simulink model "sim1S"  (R2024a)
settings: Solver=VariableStepAuto  StartTime=0.0  StopTime=500  RelTol=1e-3
values from neighbouring files (symbols this model uses):
  den = cell2mat(den)    [sim1M.m]
  den_pp = cell2mat(den_pp)    [sim1M.m]
  den_proces = cell2mat(den_proces)    [sim1M.m]
  Kr = -0.33    [sim1M.m]    (also in sim2M.m = 1/(C*inv(B*Kn-A)*B))
  num = cell2mat(num)    [sim1M.m]
  num_pp = cell2mat(num_pp)    [sim1M.m]
  num_proces = cell2mat(num_proces)    [sim1M.m]
(part 1 of 3)
settings Model: Creator=grabo  LastModifiedBy=grabo
settings OptimizationCC: ReuseModelBlockBuffer=off
settings RTWCC: GPUComputeCapability=3.5

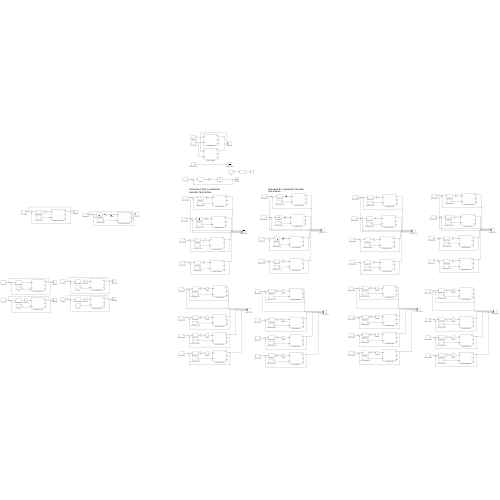
[thumbnail: Simulink's stored preview of the top-level diagram]
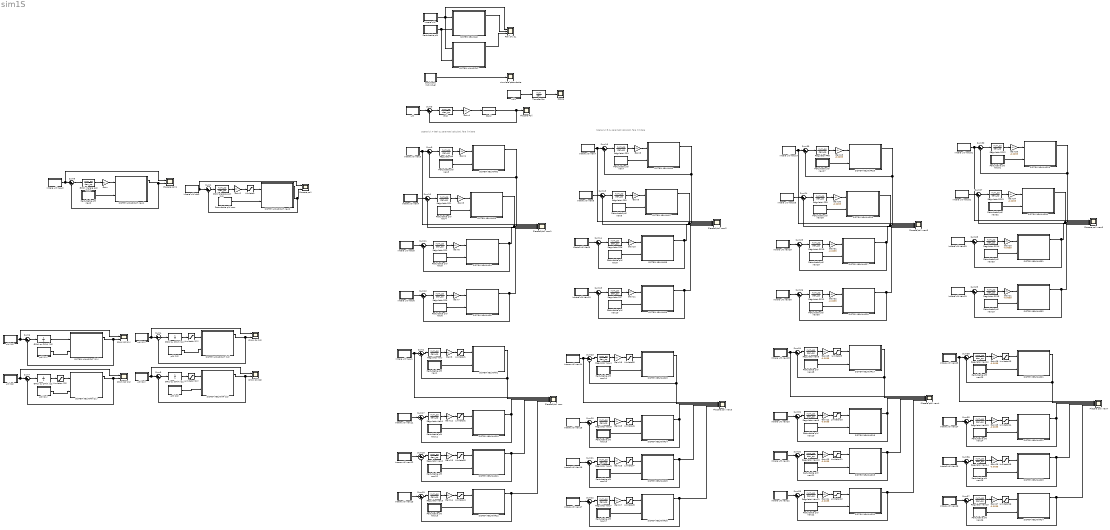
== system sim1S ==
  note: Scenariul A (G0) cu parametri calculati, fara limitare
  note: Scenariul B cu parametri calculati, fara limitare
  CMVK SL (11) : Scope  NumInputPorts=2
  CMVK SL (12) : Scope  NumInputPorts=2
  CMVK SN (21) : Scope  NumInputPorts=2
  CMVK SN (22) : Scope  NumInputPorts=2
  GR(s) cu CMVK (11) : TransferFcn  Numerator=1  Denominator=1
  GR(s) cu CMVK (12) : TransferFcn  Numerator=1  Denominator=1
  GR(s) cu CMVK (21) : TransferFcn  Numerator=1  Denominator=1
  GR(s) cu CMVK (22) : TransferFcn  Numerator=1  Denominator=1
  GR(s) plasare poli (12) : TransferFcn  Numerator=num_pp  Denominator=den_pp
  GR(s) plasare poli (12)1 : TransferFcn  Numerator=num_pp  Denominator=den_pp
  Gain{,1..18} (19 alike) : Gain  Gain=Kr
  Gain{19..34} (16 alike) : Gain  Gain=-0.0035
  Gp(s) : TransferFcn  Numerator=num_proces  Denominator=den_proces
  Gr(s) : TransferFcn  Numerator=num_pp  Denominator=den_pp
  Intrare u(t) : Subsystem  mask{With_u=1, Gref=80}
      mask prompts: With_u "With_u ="; Gref "Gref ="
  Intrare u(t) new : Subsystem  mask{With_u=1, Gref=80}
      mask prompts: With_u "With_u ="; Gref "Gref ="
  Intrare u(t) new1 : Subsystem  mask{With_u=1, Gref=80}
      mask prompts: With_u "With_u ="; Gref "Gref ="
  Intrare u(t) new10 : Subsystem  mask{With_u=1, Gref=80}
      mask prompts: With_u "With_u ="; Gref "Gref ="
  Intrare u(t) new11 : Subsystem  mask{With_u=1, Gref=80}
      mask prompts: With_u "With_u ="; Gref "Gref ="
  Intrare u(t) new12 : Subsystem  mask{With_u=1, Gref=80}
      mask prompts: With_u "With_u ="; Gref "Gref ="
  Intrare u(t) new13 : Subsystem  mask{With_u=1, Gref=80}
      mask prompts: With_u "With_u ="; Gref "Gref ="
  Intrare u(t) new14 : Subsystem  mask{With_u=1, Gref=80}
      mask prompts: With_u "With_u ="; Gref "Gref ="
  Intrare u(t) new15 : Subsystem  mask{With_u=1, Gref=80}
      mask prompts: With_u "With_u ="; Gref "Gref ="
  Intrare u(t) new16 : Subsystem  mask{With_u=1, Gref=80}
      mask prompts: With_u "With_u ="; Gref "Gref ="
  Intrare u(t) new17 : Subsystem  mask{With_u=1, Gref=80}
      mask prompts: With_u "With_u ="; Gref "Gref ="
  Intrare u(t) new18 : Subsystem  mask{With_u=1, Gref=80}
      mask prompts: With_u "With_u ="; Gref "Gref ="
  Intrare u(t) new19 : Subsystem  mask{With_u=1, Gref=80}
      mask prompts: With_u "With_u ="; Gref "Gref ="
  Intrare u(t) new2 : Subsystem  mask{With_u=1, Gref=80}
      mask prompts: With_u "With_u ="; Gref "Gref ="
  Intrare u(t) new20 : Subsystem  mask{With_u=1, Gref=80}
      mask prompts: With_u "With_u ="; Gref "Gref ="
  Intrare u(t) new21 : Subsystem  mask{With_u=1, Gref=80}
      mask prompts: With_u "With_u ="; Gref "Gref ="
  Intrare u(t) new22 : Subsystem  mask{With_u=1, Gref=80}
      mask prompts: With_u "With_u ="; Gref "Gref ="
  Intrare u(t) new23 : Subsystem  mask{With_u=1, Gref=80}
      mask prompts: With_u "With_u ="; Gref "Gref ="
  Intrare u(t) new24 : Subsystem  mask{With_u=1, Gref=80}
      mask prompts: With_u "With_u ="; Gref "Gref ="
  Intrare u(t) new25 : Subsystem  mask{With_u=1, Gref=80}
      mask prompts: With_u "With_u ="; Gref "Gref ="
  Intrare u(t) new26 : Subsystem  mask{With_u=1, Gref=80}
      mask prompts: With_u "With_u ="; Gref "Gref ="
  Intrare u(t) new27 : Subsystem  mask{With_u=1, Gref=80}
      mask prompts: With_u "With_u ="; Gref "Gref ="
  Intrare u(t) new28 : Subsystem  mask{With_u=1, Gref=80}
      mask prompts: With_u "With_u ="; Gref "Gref ="
  Intrare u(t) new29 : Subsystem  mask{With_u=1, Gref=80}
      mask prompts: With_u "With_u ="; Gref "Gref ="
  Intrare u(t) new3 : Subsystem  mask{With_u=1, Gref=80}
      mask prompts: With_u "With_u ="; Gref "Gref ="
  Intrare u(t) new30 : Subsystem  mask{With_u=1, Gref=80}
      mask prompts: With_u "With_u ="; Gref "Gref ="
  Intrare u(t) new31 : Subsystem  mask{With_u=1, Gref=80}
      mask prompts: With_u "With_u ="; Gref "Gref ="
  Intrare u(t) new32 : Subsystem  mask{With_u=1, Gref=80}
      mask prompts: With_u "With_u ="; Gref "Gref ="
  Intrare u(t) new33 : Subsystem  mask{With_u=1, Gref=80}
      mask prompts: With_u "With_u ="; Gref "Gref ="
  Intrare u(t) new4 : Subsystem  mask{With_u=1, Gref=80}
      mask prompts: With_u "With_u ="; Gref "Gref ="
  Intrare u(t) new5 : Subsystem  mask{With_u=1, Gref=80}
      mask prompts: With_u "With_u ="; Gref "Gref ="
  Intrare u(t) new6 : Subsystem  mask{With_u=1, Gref=80}
      mask prompts: With_u "With_u ="; Gref "Gref ="
  Intrare u(t) new7 : Subsystem  mask{With_u=1, Gref=80}
      mask prompts: With_u "With_u ="; Gref "Gref ="
  Intrare u(t) new8 : Subsystem  mask{With_u=1, Gref=80}
      mask prompts: With_u "With_u ="; Gref "Gref ="
  Intrare u(t) new9 : Subsystem  mask{With_u=1, Gref=80}
      mask prompts: With_u "With_u ="; Gref "Gref ="
  Limitator{,1..16} (17 alike) : Saturate  UpperLimit=500  LowerLimit=0
  Limitator (12) : Saturate  UpperLimit=500  LowerLimit=0
  Limitator (21) : Saturate  UpperLimit=500  LowerLimit=0
  Limitator (22) : Saturate  UpperLimit=500  LowerLimit=0
  Perturbatie p(t) : Subsystem  mask{Dg=100*10^3, Ag=0.8, tgM=40, With_p=1}
      mask prompts: Dg "Dg ="; Ag "Ag ="; tgM "tgM ="; With_p "With_p ="
  Perturbatie p(t) new : Subsystem  mask{Dg=100000, Ag=0.8, tgM=40, With_p=0}
      mask prompts: Dg "Dg ="; Ag "Ag ="; tgM "tgM ="; With_p "With_p ="
  Perturbatie p(t) new1 : Subsystem  mask{Dg=40*10^4, Ag=0.8, tgM=40, With_p=0}
      mask prompts: Dg "Dg ="; Ag "Ag ="; tgM "tgM ="; With_p "With_p ="
  Perturbatie p(t) new10 : Subsystem  mask{Dg=100*10^3, Ag=0.8, tgM=40, With_p=1}
      mask prompts: Dg "Dg ="; Ag "Ag ="; tgM "tgM ="; With_p "With_p ="
  Perturbatie p(t) new11 : Subsystem  mask{Dg=40*10^4, Ag=0.8, tgM=40, With_p=0}
      mask prompts: Dg "Dg ="; Ag "Ag ="; tgM "tgM ="; With_p "With_p ="
  Perturbatie p(t) new12 : Subsystem  mask{Dg=40*10^4, Ag=0.8, tgM=40, With_p=0}
      mask prompts: Dg "Dg ="; Ag "Ag ="; tgM "tgM ="; With_p "With_p ="
  Perturbatie p(t) new13 : Subsystem  mask{Dg=40*10^4, Ag=0.8, tgM=40, With_p=0}
      mask prompts: Dg "Dg ="; Ag "Ag ="; tgM "tgM ="; With_p "With_p ="
  Perturbatie p(t) new14 : Subsystem  mask{Dg=10*10^4, Ag=0.8, tgM=40, With_p=1}
      mask prompts: Dg "Dg ="; Ag "Ag ="; tgM "tgM ="; With_p "With_p ="
  Perturbatie p(t) new15 : Subsystem  mask{Dg=40*10^4, Ag=0.8, tgM=40, With_p=1}
      mask prompts: Dg "Dg ="; Ag "Ag ="; tgM "tgM ="; With_p "With_p ="
  Perturbatie p(t) new16 : Subsystem  mask{Dg=70*10^4, Ag=0.8, tgM=40, With_p=1}
      mask prompts: Dg "Dg ="; Ag "Ag ="; tgM "tgM ="; With_p "With_p ="
  Perturbatie p(t) new17 : Subsystem  mask{Dg=100*10^4, Ag=0.8, tgM=40, With_p=1}
      mask prompts: Dg "Dg ="; Ag "Ag ="; tgM "tgM ="; With_p "With_p ="
  Perturbatie p(t) new18 : Subsystem  mask{Dg=40*10^4, Ag=0.8, tgM=40, With_p=0}
      mask prompts: Dg "Dg ="; Ag "Ag ="; tgM "tgM ="; With_p "With_p ="
  Perturbatie p(t) new19 : Subsystem  mask{Dg=100*10^3, Ag=0.8, tgM=40, With_p=1}
      mask prompts: Dg "Dg ="; Ag "Ag ="; tgM "tgM ="; With_p "With_p ="
  Perturbatie p(t) new2 : Subsystem  mask{Dg=10*10^3, Ag=0.8, tgM=40, With_p=0}
      mask prompts: Dg "Dg ="; Ag "Ag ="; tgM "tgM ="; With_p "With_p ="
  Perturbatie p(t) new20 : Subsystem  mask{Dg=40*10^4, Ag=0.8, tgM=40, With_p=0}
      mask prompts: Dg "Dg ="; Ag "Ag ="; tgM "tgM ="; With_p "With_p ="
  Perturbatie p(t) new21 : Subsystem  mask{Dg=40*10^4, Ag=0.8, tgM=40, With_p=0}
      mask prompts: Dg "Dg ="; Ag "Ag ="; tgM "tgM ="; With_p "With_p ="
  Perturbatie p(t) new22 : Subsystem  mask{Dg=40*10^4, Ag=0.8, tgM=40, With_p=0}
      mask prompts: Dg "Dg ="; Ag "Ag ="; tgM "tgM ="; With_p "With_p ="
  Perturbatie p(t) new23 : Subsystem  mask{Dg=10*10^4, Ag=0.8, tgM=40, With_p=1}
      mask prompts: Dg "Dg ="; Ag "Ag ="; tgM "tgM ="; With_p "With_p ="
  Perturbatie p(t) new24 : Subsystem  mask{Dg=40*10^4, Ag=0.8, tgM=40, With_p=1}
      mask prompts: Dg "Dg ="; Ag "Ag ="; tgM "tgM ="; With_p "With_p ="
  Perturbatie p(t) new25 : Subsystem  mask{Dg=70*10^4, Ag=0.8, tgM=40, With_p=1}
      mask prompts: Dg "Dg ="; Ag "Ag ="; tgM "tgM ="; With_p "With_p ="
  Perturbatie p(t) new26 : Subsystem  mask{Dg=100*10^4, Ag=0.8, tgM=40, With_p=1}
      mask prompts: Dg "Dg ="; Ag "Ag ="; tgM "tgM ="; With_p "With_p ="
  Perturbatie p(t) new27 : Subsystem  mask{Dg=10*10^3, Ag=0.8, tgM=40, With_p=0}
      mask prompts: Dg "Dg ="; Ag "Ag ="; tgM "tgM ="; With_p "With_p ="
  Perturbatie p(t) new28 : Subsystem  mask{Dg=10*10^3, Ag=0.8, tgM=40, With_p=0}
      mask prompts: Dg "Dg ="; Ag "Ag ="; tgM "tgM ="; With_p "With_p ="
  Perturbatie p(t) new29 : Subsystem  mask{Dg=10*10^3, Ag=0.8, tgM=40, With_p=0}
      mask prompts: Dg "Dg ="; Ag "Ag ="; tgM "tgM ="; With_p "With_p ="
  Perturbatie p(t) new3 : Subsystem  mask{Dg=10*10^3, Ag=0.8, tgM=40, With_p=0}
      mask prompts: Dg "Dg ="; Ag "Ag ="; tgM "tgM ="; With_p "With_p ="
  Perturbatie p(t) new30 : Subsystem  mask{Dg=10*10^3, Ag=0.8, tgM=40, With_p=0}
      mask prompts: Dg "Dg ="; Ag "Ag ="; tgM "tgM ="; With_p "With_p ="
  Perturbatie p(t) new31 : Subsystem  mask{Dg=10*10^3, Ag=0.8, tgM=40, With_p=1}
      mask prompts: Dg "Dg ="; Ag "Ag ="; tgM "tgM ="; With_p "With_p ="
  Perturbatie p(t) new32 : Subsystem  mask{Dg=40*10^3, Ag=0.8, tgM=40, With_p=1}
      mask prompts: Dg "Dg ="; Ag "Ag ="; tgM "tgM ="; With_p "With_p ="
  Perturbatie p(t) new33 : Subsystem  mask{Dg=70*10^3, Ag=0.8, tgM=40, With_p=1}
      mask prompts: Dg "Dg ="; Ag "Ag ="; tgM "tgM ="; With_p "With_p ="
  Perturbatie p(t) new4 : Subsystem  mask{Dg=10*10^3, Ag=0.8, tgM=40, With_p=0}
      mask prompts: Dg "Dg ="; Ag "Ag ="; tgM "tgM ="; With_p "With_p ="
  Perturbatie p(t) new5 : Subsystem  mask{Dg=10*10^3, Ag=0.8, tgM=40, With_p=0}
      mask prompts: Dg "Dg ="; Ag "Ag ="; tgM "tgM ="; With_p "With_p ="
  Perturbatie p(t) new6 : Subsystem  mask{Dg=10*10^3, Ag=0.8, tgM=40, With_p=0}
      mask prompts: Dg "Dg ="; Ag "Ag ="; tgM "tgM ="; With_p "With_p ="
  Perturbatie p(t) new7 : Subsystem  mask{Dg=10*10^3, Ag=0.8, tgM=40, With_p=1}
      mask prompts: Dg "Dg ="; Ag "Ag ="; tgM "tgM ="; With_p "With_p ="
  Perturbatie p(t) new8 : Subsystem  mask{Dg=40*10^3, Ag=0.8, tgM=40, With_p=1}
      mask prompts: Dg "Dg ="; Ag "Ag ="; tgM "tgM ="; With_p "With_p ="
  Perturbatie p(t) new9 : Subsystem  mask{Dg=70*10^3, Ag=0.8, tgM=40, With_p=1}
      mask prompts: Dg "Dg ="; Ag "Ag ="; tgM "tgM ="; With_p "With_p ="
  Plasare Poli : Scope
  Plasare poli : Scope  NumInputPorts=2
  Plasare poli new{,1..7} (8 alike) : Scope  NumInputPorts=5
  Plasare poli1 : Scope  NumInputPorts=2
  "Ref, SN, SL" : Scope  NumInputPorts=3
  Regulator PP{,1..15} (16 alike) : TransferFcn  Numerator=num_pp  Denominator=den_pp
  Regulator new{,1..15} (16 alike) : TransferFcn  Numerator=num_pp  Denominator=den_pp
  SISTEM LINIARIZAT : Subsystem  mask{V=120, Ag=0.8, tgM=40, Xb=0.0054, Gb=80, p1=0.019, p2=0.021, p3=10.19*10^(-6), n=0.177, G0=300}
      mask prompts: V "V ="; Ag "Ag ="; tgM "tgM ="; Xb "Xb ="; Gb "Gb ="; p1 "p1 ="; p2 "p2 ="; p3 "p3 ="; n "n ="; G0 "G0 ="
  SISTEM LINIARIZAT (11) : Subsystem  mask{V=120, Ag=0.8, tgM=40, Xb=0.0054, Gb=80, p1=0.019, p2=0.021, p3=10.19*10^(-6), n=0.177, G0=150}
      mask prompts: V "V ="; Ag "Ag ="; tgM "tgM ="; Xb "Xb ="; Gb "Gb ="; p1 "p1 ="; p2 "p2 ="; p3 "p3 ="; n "n ="; G0 "G0 ="
  SISTEM LINIARIZAT (12) : Subsystem  mask{V=120, Ag=0.8, tgM=40, Xb=0.0054, Gb=80, p1=0.019, p2=0.021, p3=10.19*10^(-6), n=0.177, G0=150}
      mask prompts: V "V ="; Ag "Ag ="; tgM "tgM ="; Xb "Xb ="; Gb "Gb ="; p1 "p1 ="; p2 "p2 ="; p3 "p3 ="; n "n ="; G0 "G0 ="
  SISTEM LINIARIZAT new1 : Subsystem  mask{V=120, Ag=0.8, tgM=40, Xb=0.0054, Gb=80, p1=0.019, p2=0.021, p3=10.19*10^(-6), n=0.177, G0=150}
      mask prompts: V "V ="; Ag "Ag ="; tgM "tgM ="; Xb "Xb ="; Gb "Gb ="; p1 "p1 ="; p2 "p2 ="; p3 "p3 ="; n "n ="; G0 "G0 ="
  SISTEM LINIARIZAT new2 : Subsystem  mask{V=120, Ag=0.8, tgM=40, Xb=0.0054, Gb=80, p1=0.019, p2=0.021, p3=10.19*10^(-6), n=0.177, G0=350}
      mask prompts: V "V ="; Ag "Ag ="; tgM "tgM ="; Xb "Xb ="; Gb "Gb ="; p1 "p1 ="; p2 "p2 ="; p3 "p3 ="; n "n ="; G0 "G0 ="
  SISTEM NELINIAR : Subsystem  mask{V=120, Gb=80, p1=0.019, p2=0.021, p3=10.19*10^(-6), n=0.177, G0=300}
      mask prompts: V "V ="; Gb "Gb ="; p1 "p1 ="; p2 "p2 ="; p3 "p3 ="; n "n ="; G0 "G0 ="
  SISTEM NELINIAR (21) : Subsystem  mask{V=120, Gb=80, p1=0.019, p2=0.021, p3=10.19*10^(-6), n=0.177, G0=150}
      mask prompts: V "V ="; Gb "Gb ="; p1 "p1 ="; p2 "p2 ="; p3 "p3 ="; n "n ="; G0 "G0 ="
  SISTEM NELINIAR (22) : Subsystem  mask{V=120, Gb=80, p1=0.019, p2=0.021, p3=10.19*10^(-6), n=0.177, G0=150}
      mask prompts: V "V ="; Gb "Gb ="; p1 "p1 ="; p2 "p2 ="; p3 "p3 ="; n "n ="; G0 "G0 ="
  SISTEM NELINIAR1 : Subsystem  mask{V=120, Gb=80, p1=0.019, p2=0.021, p3=10.19*10^(-6), n=0.177, G0=150}
      mask prompts: V "V ="; Gb "Gb ="; p1 "p1 ="; p2 "p2 ="; p3 "p3 ="; n "n ="; G0 "G0 ="
  SISTEM NELINIAR10 : Subsystem  mask{V=120, Gb=80, p1=0.019, p2=0.021, p3=10.19*10^(-6), n=0.177, G0=200}
      mask prompts: V "V ="; Gb "Gb ="; p1 "p1 ="; p2 "p2 ="; p3 "p3 ="; n "n ="; G0 "G0 ="
  SISTEM NELINIAR11 : Subsystem  mask{V=120, Gb=80, p1=0.019, p2=0.021, p3=10.19*10^(-6), n=0.177, G0=250}
      mask prompts: V "V ="; Gb "Gb ="; p1 "p1 ="; p2 "p2 ="; p3 "p3 ="; n "n ="; G0 "G0 ="
  SISTEM NELINIAR12 : Subsystem  mask{V=120, Gb=80, p1=0.019, p2=0.021, p3=10.19*10^(-6), n=0.177, G0=300}
      mask prompts: V "V ="; Gb "Gb ="; p1 "p1 ="; p2 "p2 ="; p3 "p3 ="; n "n ="; G0 "G0 ="
  SISTEM NELINIAR13 : Subsystem  mask{V=120, Gb=80, p1=0.019, p2=0.021, p3=10.19*10^(-6), n=0.177, G0=150}
      mask prompts: V "V ="; Gb "Gb ="; p1 "p1 ="; p2 "p2 ="; p3 "p3 ="; n "n ="; G0 "G0 ="
  SISTEM NELINIAR14 : Subsystem  mask{V=120, Gb=80, p1=0.019, p2=0.021, p3=10.19*10^(-6), n=0.177, G0=150}
      mask prompts: V "V ="; Gb "Gb ="; p1 "p1 ="; p2 "p2 ="; p3 "p3 ="; n "n ="; G0 "G0 ="
  SISTEM NELINIAR15 : Subsystem  mask{V=120, Gb=80, p1=0.019, p2=0.021, p3=10.19*10^(-6), n=0.177, G0=150}
      mask prompts: V "V ="; Gb "Gb ="; p1 "p1 ="; p2 "p2 ="; p3 "p3 ="; n "n ="; G0 "G0 ="
  SISTEM NELINIAR16 : Subsystem  mask{V=120, Gb=80, p1=0.019, p2=0.021, p3=10.19*10^(-6), n=0.177, G0=150}
      mask prompts: V "V ="; Gb "Gb ="; p1 "p1 ="; p2 "p2 ="; p3 "p3 ="; n "n ="; G0 "G0 ="
  SISTEM NELINIAR17 : Subsystem  mask{V=120, Gb=80, p1=0.019, p2=0.021, p3=10.19*10^(-6), n=0.177, G0=150}
      mask prompts: V "V ="; Gb "Gb ="; p1 "p1 ="; p2 "p2 ="; p3 "p3 ="; n "n ="; G0 "G0 ="
  SISTEM NELINIAR18 : Subsystem  mask{V=120, Gb=80, p1=0.019, p2=0.021, p3=10.19*10^(-6), n=0.177, G0=200}
      mask prompts: V "V ="; Gb "Gb ="; p1 "p1 ="; p2 "p2 ="; p3 "p3 ="; n "n ="; G0 "G0 ="
  SISTEM NELINIAR19 : Subsystem  mask{V=120, Gb=80, p1=0.019, p2=0.021, p3=10.19*10^(-6), n=0.177, G0=250}
      mask prompts: V "V ="; Gb "Gb ="; p1 "p1 ="; p2 "p2 ="; p3 "p3 ="; n "n ="; G0 "G0 ="
  SISTEM NELINIAR2 : Subsystem  mask{V=120, Gb=80, p1=0.019, p2=0.021, p3=10.19*10^(-6), n=0.177, G0=150}
      mask prompts: V "V ="; Gb "Gb ="; p1 "p1 ="; p2 "p2 ="; p3 "p3 ="; n "n ="; G0 "G0 ="
  SISTEM NELINIAR20 : Subsystem  mask{V=120, Gb=80, p1=0.019, p2=0.021, p3=10.19*10^(-6), n=0.177, G0=300}
      mask prompts: V "V ="; Gb "Gb ="; p1 "p1 ="; p2 "p2 ="; p3 "p3 ="; n "n ="; G0 "G0 ="
  SISTEM NELINIAR21 : Subsystem  mask{V=120, Gb=80, p1=0.019, p2=0.021, p3=10.19*10^(-6), n=0.177, G0=150}
      mask prompts: V "V ="; Gb "Gb ="; p1 "p1 ="; p2 "p2 ="; p3 "p3 ="; n "n ="; G0 "G0 ="
  SISTEM NELINIAR22 : Subsystem  mask{V=120, Gb=80, p1=0.019, p2=0.021, p3=10.19*10^(-6), n=0.177, G0=150}
      mask prompts: V "V ="; Gb "Gb ="; p1 "p1 ="; p2 "p2 ="; p3 "p3 ="; n "n ="; G0 "G0 ="
  SISTEM NELINIAR23 : Subsystem  mask{V=120, Gb=80, p1=0.019, p2=0.021, p3=10.19*10^(-6), n=0.177, G0=150}
      mask prompts: V "V ="; Gb "Gb ="; p1 "p1 ="; p2 "p2 ="; p3 "p3 ="; n "n ="; G0 "G0 ="
  SISTEM NELINIAR24 : Subsystem  mask{V=120, Gb=80, p1=0.019, p2=0.021, p3=10.19*10^(-6), n=0.177, G0=150}
      mask prompts: V "V ="; Gb "Gb ="; p1 "p1 ="; p2 "p2 ="; p3 "p3 ="; n "n ="; G0 "G0 ="
  SISTEM NELINIAR25 : Subsystem  mask{V=120, Gb=80, p1=0.019, p2=0.021, p3=10.19*10^(-6), n=0.177, G0=150}
      mask prompts: V "V ="; Gb "Gb ="; p1 "p1 ="; p2 "p2 ="; p3 "p3 ="; n "n ="; G0 "G0 ="
  SISTEM NELINIAR26 : Subsystem  mask{V=120, Gb=80, p1=0.019, p2=0.021, p3=10.19*10^(-6), n=0.177, G0=200}
      mask prompts: V "V ="; Gb "Gb ="; p1 "p1 ="; p2 "p2 ="; p3 "p3 ="; n "n ="; G0 "G0 ="
  SISTEM NELINIAR27 : Subsystem  mask{V=120, Gb=80, p1=0.019, p2=0.021, p3=10.19*10^(-6), n=0.177, G0=250}
      mask prompts: V "V ="; Gb "Gb ="; p1 "p1 ="; p2 "p2 ="; p3 "p3 ="; n "n ="; G0 "G0 ="
  SISTEM NELINIAR28 : Subsystem  mask{V=120, Gb=80, p1=0.019, p2=0.021, p3=10.19*10^(-6), n=0.177, G0=300}
      mask prompts: V "V ="; Gb "Gb ="; p1 "p1 ="; p2 "p2 ="; p3 "p3 ="; n "n ="; G0 "G0 ="
  SISTEM NELINIAR29 : Subsystem  mask{V=120, Gb=80, p1=0.019, p2=0.021, p3=10.19*10^(-6), n=0.177, G0=150}
      mask prompts: V "V ="; Gb "Gb ="; p1 "p1 ="; p2 "p2 ="; p3 "p3 ="; n "n ="; G0 "G0 ="
  SISTEM NELINIAR3 : Subsystem  mask{V=120, Gb=80, p1=0.019, p2=0.021, p3=10.19*10^(-6), n=0.177, G0=200}
      mask prompts: V "V ="; Gb "Gb ="; p1 "p1 ="; p2 "p2 ="; p3 "p3 ="; n "n ="; G0 "G0 ="
  SISTEM NELINIAR30 : Subsystem  mask{V=120, Gb=80, p1=0.019, p2=0.021, p3=10.19*10^(-6), n=0.177, G0=200}
      mask prompts: V "V ="; Gb "Gb ="; p1 "p1 ="; p2 "p2 ="; p3 "p3 ="; n "n ="; G0 "G0 ="
  SISTEM NELINIAR31 : Subsystem  mask{V=120, Gb=80, p1=0.019, p2=0.021, p3=10.19*10^(-6), n=0.177, G0=250}
      mask prompts: V "V ="; Gb "Gb ="; p1 "p1 ="; p2 "p2 ="; p3 "p3 ="; n "n ="; G0 "G0 ="
  SISTEM NELINIAR32 : Subsystem  mask{V=120, Gb=80, p1=0.019, p2=0.021, p3=10.19*10^(-6), n=0.177, G0=300}
      mask prompts: V "V ="; Gb "Gb ="; p1 "p1 ="; p2 "p2 ="; p3 "p3 ="; n "n ="; G0 "G0 ="
  SISTEM NELINIAR4 : Subsystem  mask{V=120, Gb=80, p1=0.019, p2=0.021, p3=10.19*10^(-6), n=0.177, G0=250}
      mask prompts: V "V ="; Gb "Gb ="; p1 "p1 ="; p2 "p2 ="; p3 "p3 ="; n "n ="; G0 "G0 ="
  SISTEM NELINIAR5 : Subsystem  mask{V=120, Gb=80, p1=0.019, p2=0.021, p3=10.19*10^(-6), n=0.177, G0=300}
      mask prompts: V "V ="; Gb "Gb ="; p1 "p1 ="; p2 "p2 ="; p3 "p3 ="; n "n ="; G0 "G0 ="
  SISTEM NELINIAR6 : Subsystem  mask{V=120, Gb=80, p1=0.019, p2=0.021, p3=10.19*10^(-6), n=0.177, G0=150}
      mask prompts: V "V ="; Gb "Gb ="; p1 "p1 ="; p2 "p2 ="; p3 "p3 ="; n "n ="; G0 "G0 ="
  SISTEM NELINIAR7 : Subsystem  mask{V=120, Gb=80, p1=0.019, p2=0.021, p3=10.19*10^(-6), n=0.177, G0=200}
      mask prompts: V "V ="; Gb "Gb ="; p1 "p1 ="; p2 "p2 ="; p3 "p3 ="; n "n ="; G0 "G0 ="
  SISTEM NELINIAR8 : Subsystem  mask{V=120, Gb=80, p1=0.019, p2=0.021, p3=10.19*10^(-6), n=0.177, G0=250}
      mask prompts: V "V ="; Gb "Gb ="; p1 "p1 ="; p2 "p2 ="; p3 "p3 ="; n "n ="; G0 "G0 ="
  SISTEM NELINIAR9 : Subsystem  mask{V=120, Gb=80, p1=0.019, p2=0.021, p3=10.19*10^(-6), n=0.177, G0=300}
      mask prompts: V "V ="; Gb "Gb ="; p1 "p1 ="; p2 "p2 ="; p3 "p3 ="; n "n ="; G0 "G0 ="
  Scope : Scope
  Sum{1..39} (39 alike) : Sum  Inputs=|+-
  Transfer Fcn : TransferFcn  Numerator=num  Denominator=den
  p(t) (11) : Subsystem  mask{Dg=100000, Ag=0.8, tgM=40, With_p=0}
      mask prompts: Dg "Dg ="; Ag "Ag ="; tgM "tgM ="; With_p "With_p ="
  p(t) (12) : Subsystem  mask{Dg=100000, Ag=0.8, tgM=40, With_p=0}
      mask prompts: Dg "Dg ="; Ag "Ag ="; tgM "tgM ="; With_p "With_p ="
  p(t) (21) : Subsystem  mask{Dg=100000, Ag=0.8, tgM=40, With_p=0}
      mask prompts: Dg "Dg ="; Ag "Ag ="; tgM "tgM ="; With_p "With_p ="
  p(t) (22) : Subsystem  mask{Dg=100000, Ag=0.8, tgM=40, With_p=0}
      mask prompts: Dg "Dg ="; Ag "Ag ="; tgM "tgM ="; With_p "With_p ="
  pertubatie individual : Subsystem  mask{Dg=10*10^3, Ag=0.8, tgM=40}
      mask prompts: Dg "Dg ="; Ag "Ag ="; tgM "tgM ="
  simulare perturbatie : Scope
  u(t) : Subsystem  mask{With_u=1, Gref=80}
      mask prompts: With_u "With_u ="; Gref "Gref ="
  u(t) (11) : Subsystem  mask{With_u=1, Gref=80}
      mask prompts: With_u "With_u ="; Gref "Gref ="
  u(t) (12) : Subsystem  mask{With_u=1, Gref=80}
      mask prompts: With_u "With_u ="; Gref "Gref ="
  u(t) (21) : Subsystem  mask{With_u=1, Gref=80}
      mask prompts: With_u "With_u ="; Gref "Gref ="
  u(t) (22) : Subsystem  mask{With_u=1, Gref=80}
      mask prompts: With_u "With_u ="; Gref "Gref ="
  u(t)1 : Subsystem  mask{With_u=1, Gref=80}
      mask prompts: With_u "With_u ="; Gref "Gref ="
  wires:
  pertubatie individual/1(p(t)) -> simulare perturbatie/1
  Intrare u(t)/1(u(t)) -> SISTEM LINIARIZAT/1(u(t)), "Ref, SN, SL"/1, SISTEM NELINIAR/1(u(t))
  Perturbatie p(t)/1(p(t)) -> SISTEM LINIARIZAT/2(p(t)), SISTEM NELINIAR/2(p(t))
  Perturbatie p(t) new/1(p(t)) -> SISTEM LINIARIZAT new2/2(p(t))
  Intrare u(t) new/1(u(t)) -> Plasare poli/1, Sum1/1
  Sum1/1 -> GR(s) plasare poli (12)/1
  Sum2/1 -> Regulator new/1
  Perturbatie p(t) new1/1(p(t)) -> SISTEM NELINIAR1/2(p(t))
  Intrare u(t) new1/1(u(t)) -> Plasare poli new/1, Sum2/1
  SISTEM NELINIAR1/1(G(t)) -> Plasare poli new/2, Sum2/2
  Sum3/1 -> Gr(s)/1
  u(t)/1(u(t)) -> Sum3/1
  Gr(s)/1 -> Gain4/1
  Gp(s)/1 -> Sum3/2, Plasare Poli/1
  Regulator new/1 -> Gain3/1
  Limitator1/1 -> SISTEM NELINIAR1/1(u(t))
  GR(s) plasare poli (12)/1 -> Gain2/1
  Limitator/1 -> SISTEM LINIARIZAT new2/1(u(t))
  u(t) (22)/1(u(t)) -> CMVK SN (22)/1, Sum5/1
  p(t) (22)/1(p(t)) -> SISTEM NELINIAR (22)/2(p(t))
  Sum4/1 -> GR(s) cu CMVK (12)/1
  Sum5/1 -> GR(s) cu CMVK (22)/1
  SISTEM NELINIAR (22)/1(G(t)) -> Sum5/2, CMVK SN (22)/2
  u(t) (12)/1(u(t)) -> CMVK SL (12)/1, Sum4/1
  SISTEM LINIARIZAT (12)/1(G(t)) -> Sum4/2, CMVK SL (12)/2
  p(t) (12)/1(p(t)) -> SISTEM LINIARIZAT (12)/2(p(t))
  GR(s) cu CMVK (12)/1 -> Limitator (12)/1
  Limitator (12)/1 -> SISTEM LINIARIZAT (12)/1(u(t))
  GR(s) cu CMVK (22)/1 -> Limitator (22)/1
  Limitator (22)/1 -> SISTEM NELINIAR (22)/1(u(t))
  GR(s) cu CMVK (11)/1 -> SISTEM LINIARIZAT (11)/1(u(t))
  Sum6/1 -> GR(s) cu CMVK (11)/1
  SISTEM LINIARIZAT (11)/1(G(t)) -> Sum6/2, CMVK SL (11)/2
  u(t) (11)/1(u(t)) -> CMVK SL (11)/1, Sum6/1
  p(t) (11)/1(p(t)) -> SISTEM LINIARIZAT (11)/2(p(t))
  Limitator (21)/1 -> SISTEM NELINIAR (21)/1(u(t))
  GR(s) cu CMVK (21)/1 -> Limitator (21)/1
  u(t) (21)/1(u(t)) -> CMVK SN (21)/1, Sum7/1
  Sum7/1 -> GR(s) cu CMVK (21)/1
  p(t) (21)/1(p(t)) -> SISTEM NELINIAR (21)/2(p(t))
  SISTEM NELINIAR (21)/1(G(t)) -> Sum7/2, CMVK SN (21)/2
  GR(s) plasare poli (12)1/1 -> Gain/1
  Intrare u(t) new2/1(u(t)) -> Plasare poli1/1, Sum8/1
  Sum8/1 -> GR(s) plasare poli (12)1/1
  SISTEM LINIARIZAT new1/1(G(t)) -> Sum8/2, Plasare poli1/2
  Perturbatie p(t) new2/1(p(t)) -> SISTEM LINIARIZAT new1/2(p(t))
  Regulator PP/1 -> Gain1/1
  Perturbatie p(t) new3/1(p(t)) -> SISTEM NELINIAR2/2(p(t))
  Intrare u(t) new3/1(u(t)) -> Plasare poli new1/1, Sum9/1
  Sum9/1 -> Regulator PP/1
  SISTEM NELINIAR2/1(G(t)) -> Sum9/2, Plasare poli new1/2
  Gain/1 -> SISTEM LINIARIZAT new1/1(u(t))
  Gain1/1 -> SISTEM NELINIAR2/1(u(t))
  Gain2/1 -> Limitator/1
  Gain3/1 -> Limitator1/1
  SISTEM LINIARIZAT new2/1(G(t)) -> Sum1/2, Plasare poli/2
  Gain4/1 -> Gp(s)/1
  SISTEM NELINIAR/1(G(t)) -> "Ref, SN, SL"/2
  SISTEM LINIARIZAT/1(G(t)) -> "Ref, SN, SL"/3
  Perturbatie p(t) new4/1(p(t)) -> SISTEM NELINIAR3/2(p(t))
  Gain5/1 -> SISTEM NELINIAR3/1(u(t))
  SISTEM NELINIAR3/1(G(t)) -> Sum10/2, Plasare poli new1/3
  Intrare u(t) new4/1(u(t)) -> Sum10/1
  Regulator PP1/1 -> Gain5/1
  Sum10/1 -> Regulator PP1/1
  Perturbatie p(t) new5/1(p(t)) -> SISTEM NELINIAR4/2(p(t))
  Gain6/1 -> SISTEM NELINIAR4/1(u(t))
  SISTEM NELINIAR4/1(G(t)) -> Plasare poli new1/4, Sum11/2
  Intrare u(t) new5/1(u(t)) -> Sum11/1
  Regulator PP2/1 -> Gain6/1
  Sum11/1 -> Regulator PP2/1
  Perturbatie p(t) new6/1(p(t)) -> SISTEM NELINIAR5/2(p(t))
  Gain7/1 -> SISTEM NELINIAR5/1(u(t))
  SISTEM NELINIAR5/1(G(t)) -> Plasare poli new1/5, Sum12/2
  Intrare u(t) new6/1(u(t)) -> Sum12/1
  Regulator PP3/1 -> Gain7/1
  Sum12/1 -> Regulator PP3/1
  Sum14/1 -> Regulator PP6/1
  Regulator PP6/1 -> Gain10/1
  SISTEM NELINIAR8/1(G(t)) -> Plasare poli new2/4, Sum14/2
  Intrare u(t) new8/1(u(t)) -> Sum13/1
  Sum13/1 -> Regulator PP5/1
  Regulator PP5/1 -> Gain9/1
  Gain9/1 -> SISTEM NELINIAR7/1(u(t))
  Perturbatie p(t) new8/1(p(t)) -> SISTEM NELINIAR7/2(p(t))
  Gain10/1 -> SISTEM NELINIAR8/1(u(t))
  Regulator PP7/1 -> Gain11/1
  Sum15/1 -> Regulator PP7/1
  Intrare u(t) new9/1(u(t)) -> Sum14/1
  Intrare u(t) new10/1(u(t)) -> Sum15/1
  Perturbatie p(t) new9/1(p(t)) -> SISTEM NELINIAR8/2(p(t))
  SISTEM NELINIAR9/1(G(t)) -> Plasare poli new2/5, Sum15/2
  Gain11/1 -> SISTEM NELINIAR9/1(u(t))
  Perturbatie p(t) new7/1(p(t)) -> SISTEM NELINIAR6/2(p(t))
  Gain8/1 -> SISTEM NELINIAR6/1(u(t))
  SISTEM NELINIAR6/1(G(t)) -> Sum16/2, Plasare poli new2/2
  Intrare u(t) new7/1(u(t)) -> Plasare poli new2/1, Sum16/1
  SISTEM NELINIAR7/1(G(t)) -> Sum13/2, Plasare poli new2/3
  Regulator PP4/1 -> Gain8/1
  Perturbatie p(t) new10/1(p(t)) -> SISTEM NELINIAR9/2(p(t))
  Sum16/1 -> Regulator PP4/1
  SISTEM NELINIAR10/1(G(t)) -> Sum17/2, Plasare poli new/3
  Regulator new1/1 -> Gain12/1
  Sum17/1 -> Regulator new1/1
  Limitator2/1 -> SISTEM NELINIAR10/1(u(t))
  Gain12/1 -> Limitator2/1
  Intrare u(t) new11/1(u(t)) -> Sum17/1
  Perturbatie p(t) new11/1(p(t)) -> SISTEM NELINIAR10/2(p(t))
  Perturbatie p(t) new12/1(p(t)) -> SISTEM NELINIAR11/2(p(t))
  Gain13/1 -> Limitator3/1
  Regulator new2/1 -> Gain13/1
  Limitator3/1 -> SISTEM NELINIAR11/1(u(t))
  Sum18/1 -> Regulator new2/1
  Intrare u(t) new12/1(u(t)) -> Sum18/1
  SISTEM NELINIAR11/1(G(t)) -> Plasare poli new/4, Sum18/2
  Perturbatie p(t) new13/1(p(t)) -> SISTEM NELINIAR12/2(p(t))
  Gain14/1 -> Limitator4/1
  Regulator new3/1 -> Gain14/1
  Limitator4/1 -> SISTEM NELINIAR12/1(u(t))
  Sum19/1 -> Regulator new3/1
  Intrare u(t) new13/1(u(t)) -> Sum19/1
  SISTEM NELINIAR12/1(G(t)) -> Plasare poli new/5, Sum19/2
  Sum22/1 -> Regulator new7/1
  Intrare u(t) new17/1(u(t)) -> Sum22/1
  Regulator new7/1 -> Gain17/1
  Gain17/1 -> Limitator8/1
  Intrare u(t) new15/1(u(t)) -> Sum20/1
  Sum20/1 -> Regulator new5/1
  Gain15/1 -> Limitator6/1
  Regulator new5/1 -> Gain15/1
  Limitator6/1 -> SISTEM NELINIAR14/1(u(t))
  SISTEM NELINIAR14/1(G(t)) -> Sum20/2, Plasare poli new3/3
  Gain16/1 -> Limitator7/1
  Intrare u(t) new16/1(u(t)) -> Sum21/1
  SISTEM NELINIAR15/1(G(t)) -> Plasare poli new3/4, Sum21/2
  Sum21/1 -> Regulator new6/1
  Limitator7/1 -> SISTEM NELINIAR15/1(u(t))
  Regulator new6/1 -> Gain16/1
  Perturbatie p(t) new17/1(p(t)) -> SISTEM NELINIAR16/2(p(t))
  SISTEM NELINIAR16/1(G(t)) -> Plasare poli new3/5, Sum22/2
  Perturbatie p(t) new15/1(p(t)) -> SISTEM NELINIAR14/2(p(t))
  SISTEM NELINIAR13/1(G(t)) -> Plasare poli new3/2, Sum23/2
  Regulator new4/1 -> Gain18/1
  Sum23/1 -> Regulator new4/1
  Limitator5/1 -> SISTEM NELINIAR13/1(u(t))
  Limitator8/1 -> SISTEM NELINIAR16/1(u(t))
  Perturbatie p(t) new16/1(p(t)) -> SISTEM NELINIAR15/2(p(t))
  Gain18/1 -> Limitator5/1
  Intrare u(t) new14/1(u(t)) -> Plasare poli new3/1, Sum23/1
  Perturbatie p(t) new14/1(p(t)) -> SISTEM NELINIAR13/2(p(t))
  Sum33/1 -> Regulator new11/1
  Intrare u(t) new22/1(u(t)) -> Sum33/1
  Perturbatie p(t) new22/1(p(t)) -> SISTEM NELINIAR20/2(p(t))
  Perturbatie p(t) new20/1(p(t)) -> SISTEM NELINIAR18/2(p(t))
  Intrare u(t) new20/1(u(t)) -> Sum31/1
  Sum31/1 -> Regulator new9/1
  Regulator new9/1 -> Gain22/1
  Limitator10/1 -> SISTEM NELINIAR18/1(u(t))
  SISTEM NELINIAR18/1(G(t)) -> Sum31/2, Plasare poli new4/3
  Regulator new12/1 -> Gain28/1
  SISTEM NELINIAR21/1(G(t)) -> Plasare poli new7/2, Sum38/2
  Sum38/1 -> Regulator new12/1
  Limitator13/1 -> SISTEM NELINIAR21/1(u(t))
  Perturbatie p(t) new25/1(p(t)) -> SISTEM NELINIAR23/2(p(t))
  Limitator16/1 -> SISTEM NELINIAR24/1(u(t))
  Gain28/1 -> Limitator13/1
  Gain24/1 -> Limitator12/1
  SISTEM NELINIAR24/1(G(t)) -> Plasare poli new7/5, Sum37/2
  Perturbatie p(t) new26/1(p(t)) -> SISTEM NELINIAR24/2(p(t))
  Perturbatie p(t) new24/1(p(t)) -> SISTEM NELINIAR22/2(p(t))
  Sum36/1 -> Regulator new14/1
  Gain26/1 -> Limitator15/1
  SISTEM NELINIAR23/1(G(t)) -> Plasare poli new7/4, Sum36/2
  Intrare u(t) new25/1(u(t)) -> Sum36/1
  Limitator14/1 -> SISTEM NELINIAR22/1(u(t))
  SISTEM NELINIAR22/1(G(t)) -> Sum35/2, Plasare poli new7/3
  Regulator new13/1 -> Gain25/1
  Gain27/1 -> Limitator16/1
  Sum37/1 -> Regulator new15/1
  Intrare u(t) new24/1(u(t)) -> Sum35/1
  Gain22/1 -> Limitator10/1
  Regulator new15/1 -> Gain27/1
  Intrare u(t) new23/1(u(t)) -> Plasare poli new7/1, Sum38/1
  Perturbatie p(t) new23/1(p(t)) -> SISTEM NELINIAR21/2(p(t))
  Perturbatie p(t) new21/1(p(t)) -> SISTEM NELINIAR19/2(p(t))
  Intrare u(t) new21/1(u(t)) -> Sum32/1
  SISTEM NELINIAR19/1(G(t)) -> Plasare poli new4/4, Sum32/2
  Limitator11/1 -> SISTEM NELINIAR19/1(u(t))
  Perturbatie p(t) new19/1(p(t)) -> SISTEM NELINIAR32/2(p(t))
  Sum30/1 -> Regulator PP12/1
  Regulator PP12/1 -> Gain33/1
  Intrare u(t) new31/1(u(t)) -> Plasare poli new6/1, Sum30/1
  SISTEM NELINIAR30/1(G(t)) -> Sum27/2, Plasare poli new6/3
  Gain21/1 -> SISTEM NELINIAR32/1(u(t))
  SISTEM NELINIAR32/1(G(t)) -> Plasare poli new6/5, Sum29/2
  Gain33/1 -> SISTEM NELINIAR29/1(u(t))
  SISTEM NELINIAR29/1(G(t)) -> Sum30/2, Plasare poli new6/2
  Intrare u(t) new26/1(u(t)) -> Sum37/1
  Perturbatie p(t) new33/1(p(t)) -> SISTEM NELINIAR31/2(p(t))
  Regulator PP15/1 -> Gain21/1
  Perturbatie p(t) new32/1(p(t)) -> SISTEM NELINIAR30/2(p(t))
  Sum29/1 -> Regulator PP15/1
  Intrare u(t) new32/1(u(t)) -> Sum27/1
  Regulator new10/1 -> Gain23/1
  Regulator PP13/1 -> Gain34/1
  Sum27/1 -> Regulator PP13/1
  Regulator new11/1 -> Gain24/1
  SISTEM NELINIAR31/1(G(t)) -> Plasare poli new6/4, Sum28/2
  Regulator PP14/1 -> Gain20/1
  Intrare u(t) new19/1(u(t)) -> Sum29/1
  Sum25/1 -> Regulator PP10/1
  Regulator PP10/1 -> Gain31/1
  Intrare u(t) new28/1(u(t)) -> Sum24/1
  Sum24/1 -> Regulator PP9/1
  Regulator new14/1 -> Gain26/1
  Gain34/1 -> SISTEM NELINIAR30/1(u(t))
  Gain23/1 -> Limitator11/1
  Gain20/1 -> SISTEM NELINIAR31/1(u(t))
  Regulator PP9/1 -> Gain30/1
  Gain30/1 -> SISTEM NELINIAR26/1(u(t))
  Limitator15/1 -> SISTEM NELINIAR23/1(u(t))
  Perturbatie p(t) new28/1(p(t)) -> SISTEM NELINIAR26/2(p(t))
  Intrare u(t) new33/1(u(t)) -> Sum28/1
  SISTEM NELINIAR20/1(G(t)) -> Plasare poli new4/5, Sum33/2
  Gain31/1 -> SISTEM NELINIAR27/1(u(t))
  Regulator PP11/1 -> Gain32/1
  Sum26/1 -> Regulator PP11/1
  Intrare u(t) new29/1(u(t)) -> Sum25/1
  Intrare u(t) new30/1(u(t)) -> Sum26/1
  Perturbatie p(t) new29/1(p(t)) -> SISTEM NELINIAR27/2(p(t))
  SISTEM NELINIAR28/1(G(t)) -> Plasare poli new5/5, Sum26/2
  Perturbatie p(t) new27/1(p(t)) -> SISTEM NELINIAR25/2(p(t))
  SISTEM NELINIAR17/1(G(t)) -> Plasare poli new4/2, Sum34/2
  Perturbatie p(t) new31/1(p(t)) -> SISTEM NELINIAR29/2(p(t))
  Gain32/1 -> SISTEM NELINIAR28/1(u(t))
  Gain25/1 -> Limitator14/1
  Gain29/1 -> Limitator9/1
  SISTEM NELINIAR25/1(G(t)) -> Sum39/2, Plasare poli new5/2
  Gain19/1 -> SISTEM NELINIAR25/1(u(t))
  Intrare u(t) new27/1(u(t)) -> Plasare poli new5/1, Sum39/1
  SISTEM NELINIAR26/1(G(t)) -> Sum24/2, Plasare poli new5/3
  Regulator PP8/1 -> Gain19/1
  Sum32/1 -> Regulator new10/1
  Perturbatie p(t) new30/1(p(t)) -> SISTEM NELINIAR28/2(p(t))
  Sum39/1 -> Regulator PP8/1
  Regulator new8/1 -> Gain29/1
  Sum34/1 -> Regulator new8/1
  Limitator9/1 -> SISTEM NELINIAR17/1(u(t))
  Sum28/1 -> Regulator PP14/1
  Limitator12/1 -> SISTEM NELINIAR20/1(u(t))
  Sum35/1 -> Regulator new13/1
  Intrare u(t) new18/1(u(t)) -> Plasare poli new4/1, Sum34/1
  SISTEM NELINIAR27/1(G(t)) -> Plasare poli new5/4, Sum25/2
  Perturbatie p(t) new18/1(p(t)) -> SISTEM NELINIAR17/2(p(t))
  Transfer Fcn/1 -> Scope/1
  u(t)1/1(u(t)) -> Transfer Fcn/1

== system sim1S/Intrare u(t) ==
  Gain : Gain  Gain=With_u
  Step : Step  Time=0  After=Gref  SampleTime=0
  u(t) : Outport
  wires:
  Step/1 -> Gain/1
  Gain/1 -> u(t)/1

== system sim1S/Intrare u(t) new ==
  Gain : Gain  Gain=With_u
  Step : Step  Time=0  After=Gref  SampleTime=0
  u(t) : Outport
  wires:
  Step/1 -> Gain/1
  Gain/1 -> u(t)/1

== system sim1S/Intrare u(t) new1 ==
  Gain : Gain  Gain=With_u
  Step : Step  Time=0  After=Gref  SampleTime=0
  u(t) : Outport
  wires:
  Step/1 -> Gain/1
  Gain/1 -> u(t)/1

== system sim1S/Intrare u(t) new10 ==
  Gain : Gain  Gain=With_u
  Step : Step  Time=0  After=Gref  SampleTime=0
  u(t) : Outport
  wires:
  Step/1 -> Gain/1
  Gain/1 -> u(t)/1

== system sim1S/Intrare u(t) new11 ==
  Gain : Gain  Gain=With_u
  Step : Step  Time=0  After=Gref  SampleTime=0
  u(t) : Outport
  wires:
  Step/1 -> Gain/1
  Gain/1 -> u(t)/1

== system sim1S/Intrare u(t) new12 ==
  Gain : Gain  Gain=With_u
  Step : Step  Time=0  After=Gref  SampleTime=0
  u(t) : Outport
  wires:
  Step/1 -> Gain/1
  Gain/1 -> u(t)/1

== system sim1S/Intrare u(t) new13 ==
  Gain : Gain  Gain=With_u
  Step : Step  Time=0  After=Gref  SampleTime=0
  u(t) : Outport
  wires:
  Step/1 -> Gain/1
  Gain/1 -> u(t)/1

== system sim1S/Intrare u(t) new14 ==
  Gain : Gain  Gain=With_u
  Step : Step  Time=0  After=Gref  SampleTime=0
  u(t) : Outport
  wires:
  Step/1 -> Gain/1
  Gain/1 -> u(t)/1

== system sim1S/Intrare u(t) new15 ==
  Gain : Gain  Gain=With_u
  Step : Step  Time=0  After=Gref  SampleTime=0
  u(t) : Outport
  wires:
  Step/1 -> Gain/1
  Gain/1 -> u(t)/1

== system sim1S/Intrare u(t) new16 ==
  Gain : Gain  Gain=With_u
  Step : Step  Time=0  After=Gref  SampleTime=0
  u(t) : Outport
  wires:
  Step/1 -> Gain/1
  Gain/1 -> u(t)/1

== system sim1S/Intrare u(t) new17 ==
  Gain : Gain  Gain=With_u
  Step : Step  Time=0  After=Gref  SampleTime=0
  u(t) : Outport
  wires:
  Step/1 -> Gain/1
  Gain/1 -> u(t)/1

== system sim1S/Intrare u(t) new18 ==
  Gain : Gain  Gain=With_u
  Step : Step  Time=0  After=Gref  SampleTime=0
  u(t) : Outport
  wires:
  Step/1 -> Gain/1
  Gain/1 -> u(t)/1

== system sim1S/Intrare u(t) new19 ==
  Gain : Gain  Gain=With_u
  Step : Step  Time=0  After=Gref  SampleTime=0
  u(t) : Outport
  wires:
  Step/1 -> Gain/1
  Gain/1 -> u(t)/1

== system sim1S/Intrare u(t) new2 ==
  Gain : Gain  Gain=With_u
  Step : Step  Time=0  After=Gref  SampleTime=0
  u(t) : Outport
  wires:
  Step/1 -> Gain/1
  Gain/1 -> u(t)/1

== system sim1S/Intrare u(t) new20 ==
  Gain : Gain  Gain=With_u
  Step : Step  Time=0  After=Gref  SampleTime=0
  u(t) : Outport
  wires:
  Step/1 -> Gain/1
  Gain/1 -> u(t)/1

== system sim1S/Intrare u(t) new21 ==
  Gain : Gain  Gain=With_u
  Step : Step  Time=0  After=Gref  SampleTime=0
  u(t) : Outport
  wires:
  Step/1 -> Gain/1
  Gain/1 -> u(t)/1

== system sim1S/Intrare u(t) new22 ==
  Gain : Gain  Gain=With_u
  Step : Step  Time=0  After=Gref  SampleTime=0
  u(t) : Outport
  wires:
  Step/1 -> Gain/1
  Gain/1 -> u(t)/1

== system sim1S/Intrare u(t) new23 ==
  Gain : Gain  Gain=With_u
  Step : Step  Time=0  After=Gref  SampleTime=0
  u(t) : Outport
  wires:
  Step/1 -> Gain/1
  Gain/1 -> u(t)/1

== system sim1S/Intrare u(t) new24 ==
  Gain : Gain  Gain=With_u
  Step : Step  Time=0  After=Gref  SampleTime=0
  u(t) : Outport
  wires:
  Step/1 -> Gain/1
  Gain/1 -> u(t)/1

== system sim1S/Intrare u(t) new25 ==
  Gain : Gain  Gain=With_u
  Step : Step  Time=0  After=Gref  SampleTime=0
  u(t) : Outport
  wires:
  Step/1 -> Gain/1
  Gain/1 -> u(t)/1

== system sim1S/Intrare u(t) new26 ==
  Gain : Gain  Gain=With_u
  Step : Step  Time=0  After=Gref  SampleTime=0
  u(t) : Outport
  wires:
  Step/1 -> Gain/1
  Gain/1 -> u(t)/1

== system sim1S/Intrare u(t) new27 ==
  Gain : Gain  Gain=With_u
  Step : Step  Time=0  After=Gref  SampleTime=0
  u(t) : Outport
  wires:
  Step/1 -> Gain/1
  Gain/1 -> u(t)/1

== system sim1S/Intrare u(t) new28 ==
  Gain : Gain  Gain=With_u
  Step : Step  Time=0  After=Gref  SampleTime=0
  u(t) : Outport
  wires:
  Step/1 -> Gain/1
  Gain/1 -> u(t)/1

== system sim1S/Intrare u(t) new29 ==
  Gain : Gain  Gain=With_u
  Step : Step  Time=0  After=Gref  SampleTime=0
  u(t) : Outport
  wires:
  Step/1 -> Gain/1
  Gain/1 -> u(t)/1

== system sim1S/Intrare u(t) new3 ==
  Gain : Gain  Gain=With_u
  Step : Step  Time=0  After=Gref  SampleTime=0
  u(t) : Outport
  wires:
  Step/1 -> Gain/1
  Gain/1 -> u(t)/1

== system sim1S/Intrare u(t) new30 ==
  Gain : Gain  Gain=With_u
  Step : Step  Time=0  After=Gref  SampleTime=0
  u(t) : Outport
  wires:
  Step/1 -> Gain/1
  Gain/1 -> u(t)/1

== system sim1S/Intrare u(t) new31 ==
  Gain : Gain  Gain=With_u
  Step : Step  Time=0  After=Gref  SampleTime=0
  u(t) : Outport
  wires:
  Step/1 -> Gain/1
  Gain/1 -> u(t)/1

== system sim1S/Intrare u(t) new32 ==
  Gain : Gain  Gain=With_u
  Step : Step  Time=0  After=Gref  SampleTime=0
  u(t) : Outport
  wires:
  Step/1 -> Gain/1
  Gain/1 -> u(t)/1

== system sim1S/Intrare u(t) new33 ==
  Gain : Gain  Gain=With_u
  Step : Step  Time=0  After=Gref  SampleTime=0
  u(t) : Outport
  wires:
  Step/1 -> Gain/1
  Gain/1 -> u(t)/1

== system sim1S/Intrare u(t) new4 ==
  Gain : Gain  Gain=With_u
  Step : Step  Time=0  After=Gref  SampleTime=0
  u(t) : Outport
  wires:
  Step/1 -> Gain/1
  Gain/1 -> u(t)/1

== system sim1S/Intrare u(t) new5 ==
  Gain : Gain  Gain=With_u
  Step : Step  Time=0  After=Gref  SampleTime=0
  u(t) : Outport
  wires:
  Step/1 -> Gain/1
  Gain/1 -> u(t)/1

== system sim1S/Intrare u(t) new6 ==
  Gain : Gain  Gain=With_u
  Step : Step  Time=0  After=Gref  SampleTime=0
  u(t) : Outport
  wires:
  Step/1 -> Gain/1
  Gain/1 -> u(t)/1

== system sim1S/Intrare u(t) new7 ==
  Gain : Gain  Gain=With_u
  Step : Step  Time=0  After=Gref  SampleTime=0
  u(t) : Outport
  wires:
  Step/1 -> Gain/1
  Gain/1 -> u(t)/1

== system sim1S/Intrare u(t) new8 ==
  Gain : Gain  Gain=With_u
  Step : Step  Time=0  After=Gref  SampleTime=0
  u(t) : Outport
  wires:
  Step/1 -> Gain/1
  Gain/1 -> u(t)/1

== system sim1S/Intrare u(t) new9 ==
  Gain : Gain  Gain=With_u
  Step : Step  Time=0  After=Gref  SampleTime=0
  u(t) : Outport
  wires:
  Step/1 -> Gain/1
  Gain/1 -> u(t)/1

== system sim1S/Perturbatie p(t) ==
  Clock1 : Clock
  Constant1 : Constant  Value=Dg
  Constant2 : Constant  Value=Ag
  Constant3 : Constant  Value=-1/tgM
  Constant4 : Constant  Value=1/(tgM^2)
  Gain : Gain  Gain=With_p
  Math Function : Math  SignedPower=on
  Product1 : Product
  Product3 : Product  Inputs=5
  p(t) : Outport
  wires:
  Clock1/1 -> Product3/5, Product1/1
  Constant3/1 -> Product1/2
  Product1/1 -> Math Function/1
  Constant4/1 -> Product3/4
  Constant1/1 -> Product3/1
  Constant2/1 -> Product3/2
  Math Function/1 -> Product3/3
  Product3/1 -> Gain/1
  Gain/1 -> p(t)/1

== system sim1S/Perturbatie p(t) new ==
  Clock1 : Clock
  Constant1 : Constant  Value=Dg
  Constant2 : Constant  Value=Ag
  Constant3 : Constant  Value=-1/tgM
  Constant4 : Constant  Value=1/(tgM^2)
  Gain : Gain  Gain=With_p
  Math Function : Math  SignedPower=on
  Product1 : Product
  Product3 : Product  Inputs=5
  p(t) : Outport
  wires:
  Clock1/1 -> Product3/5, Product1/1
  Constant3/1 -> Product1/2
  Product1/1 -> Math Function/1
  Constant4/1 -> Product3/4
  Constant1/1 -> Product3/1
  Constant2/1 -> Product3/2
  Math Function/1 -> Product3/3
  Product3/1 -> Gain/1
  Gain/1 -> p(t)/1

== system sim1S/Perturbatie p(t) new1 ==
  Clock1 : Clock
  Constant1 : Constant  Value=Dg
  Constant2 : Constant  Value=Ag
  Constant3 : Constant  Value=-1/tgM
  Constant4 : Constant  Value=1/(tgM^2)
  Gain : Gain  Gain=With_p
  Math Function : Math  SignedPower=on
  Product1 : Product
  Product3 : Product  Inputs=5
  p(t) : Outport
  wires:
  Clock1/1 -> Product3/5, Product1/1
  Constant3/1 -> Product1/2
  Product1/1 -> Math Function/1
  Constant4/1 -> Product3/4
  Constant1/1 -> Product3/1
  Constant2/1 -> Product3/2
  Math Function/1 -> Product3/3
  Product3/1 -> Gain/1
  Gain/1 -> p(t)/1

== system sim1S/Perturbatie p(t) new10 ==
  Clock1 : Clock
  Constant1 : Constant  Value=Dg
  Constant2 : Constant  Value=Ag
  Constant3 : Constant  Value=-1/tgM
  Constant4 : Constant  Value=1/(tgM^2)
  Gain : Gain  Gain=With_p
  Math Function : Math  SignedPower=on
  Product1 : Product
  Product3 : Product  Inputs=5
  p(t) : Outport
  wires:
  Clock1/1 -> Product3/5, Product1/1
  Constant3/1 -> Product1/2
  Product1/1 -> Math Function/1
  Constant4/1 -> Product3/4
  Constant1/1 -> Product3/1
  Constant2/1 -> Product3/2
  Math Function/1 -> Product3/3
  Product3/1 -> Gain/1
  Gain/1 -> p(t)/1

== system sim1S/Perturbatie p(t) new11 ==
  Clock1 : Clock
  Constant1 : Constant  Value=Dg
  Constant2 : Constant  Value=Ag
  Constant3 : Constant  Value=-1/tgM
  Constant4 : Constant  Value=1/(tgM^2)
  Gain : Gain  Gain=With_p
  Math Function : Math  SignedPower=on
  Product1 : Product
  Product3 : Product  Inputs=5
  p(t) : Outport
  wires:
  Clock1/1 -> Product3/5, Product1/1
  Constant3/1 -> Product1/2
  Product1/1 -> Math Function/1
  Constant4/1 -> Product3/4
  Constant1/1 -> Product3/1
  Constant2/1 -> Product3/2
  Math Function/1 -> Product3/3
  Product3/1 -> Gain/1
  Gain/1 -> p(t)/1

== system sim1S/Perturbatie p(t) new12 ==
  Clock1 : Clock
  Constant1 : Constant  Value=Dg
  Constant2 : Constant  Value=Ag
  Constant3 : Constant  Value=-1/tgM
  Constant4 : Constant  Value=1/(tgM^2)
  Gain : Gain  Gain=With_p
  Math Function : Math  SignedPower=on
  Product1 : Product
  Product3 : Product  Inputs=5
  p(t) : Outport
  wires:
  Clock1/1 -> Product3/5, Product1/1
  Constant3/1 -> Product1/2
  Product1/1 -> Math Function/1
  Constant4/1 -> Product3/4
  Constant1/1 -> Product3/1
  Constant2/1 -> Product3/2
  Math Function/1 -> Product3/3
  Product3/1 -> Gain/1
  Gain/1 -> p(t)/1

== system sim1S/Perturbatie p(t) new13 ==
  Clock1 : Clock
  Constant1 : Constant  Value=Dg
  Constant2 : Constant  Value=Ag
  Constant3 : Constant  Value=-1/tgM
  Constant4 : Constant  Value=1/(tgM^2)
  Gain : Gain  Gain=With_p
  Math Function : Math  SignedPower=on
  Product1 : Product
  Product3 : Product  Inputs=5
  p(t) : Outport
  wires:
  Clock1/1 -> Product3/5, Product1/1
  Constant3/1 -> Product1/2
  Product1/1 -> Math Function/1
  Constant4/1 -> Product3/4
  Constant1/1 -> Product3/1
  Constant2/1 -> Product3/2
  Math Function/1 -> Product3/3
  Product3/1 -> Gain/1
  Gain/1 -> p(t)/1

== system sim1S/Perturbatie p(t) new14 ==
  Clock1 : Clock
  Constant1 : Constant  Value=Dg
  Constant2 : Constant  Value=Ag
  Constant3 : Constant  Value=-1/tgM
  Constant4 : Constant  Value=1/(tgM^2)
  Gain : Gain  Gain=With_p
  Math Function : Math  SignedPower=on
  Product1 : Product
  Product3 : Product  Inputs=5
  p(t) : Outport
  wires:
  Clock1/1 -> Product3/5, Product1/1
  Constant3/1 -> Product1/2
  Product1/1 -> Math Function/1
  Constant4/1 -> Product3/4
  Constant1/1 -> Product3/1
  Constant2/1 -> Product3/2
  Math Function/1 -> Product3/3
  Product3/1 -> Gain/1
  Gain/1 -> p(t)/1

== system sim1S/Perturbatie p(t) new15 ==
  Clock1 : Clock
  Constant1 : Constant  Value=Dg
  Constant2 : Constant  Value=Ag
  Constant3 : Constant  Value=-1/tgM
  Constant4 : Constant  Value=1/(tgM^2)
  Gain : Gain  Gain=With_p
  Math Function : Math  SignedPower=on
  Product1 : Product
  Product3 : Product  Inputs=5
  p(t) : Outport
  wires:
  Clock1/1 -> Product3/5, Product1/1
  Constant3/1 -> Product1/2
  Product1/1 -> Math Function/1
  Constant4/1 -> Product3/4
  Constant1/1 -> Product3/1
  Constant2/1 -> Product3/2
  Math Function/1 -> Product3/3
  Product3/1 -> Gain/1
  Gain/1 -> p(t)/1

== system sim1S/Perturbatie p(t) new16 ==
  Clock1 : Clock
  Constant1 : Constant  Value=Dg
  Constant2 : Constant  Value=Ag
  Constant3 : Constant  Value=-1/tgM
  Constant4 : Constant  Value=1/(tgM^2)
  Gain : Gain  Gain=With_p
  Math Function : Math  SignedPower=on
  Product1 : Product
  Product3 : Product  Inputs=5
  p(t) : Outport
  wires:
  Clock1/1 -> Product3/5, Product1/1
  Constant3/1 -> Product1/2
  Product1/1 -> Math Function/1
  Constant4/1 -> Product3/4
  Constant1/1 -> Product3/1
  Constant2/1 -> Product3/2
  Math Function/1 -> Product3/3
  Product3/1 -> Gain/1
  Gain/1 -> p(t)/1

== system sim1S/Perturbatie p(t) new17 ==
  Clock1 : Clock
  Constant1 : Constant  Value=Dg
  Constant2 : Constant  Value=Ag
  Constant3 : Constant  Value=-1/tgM
  Constant4 : Constant  Value=1/(tgM^2)
  Gain : Gain  Gain=With_p
  Math Function : Math  SignedPower=on
  Product1 : Product
  Product3 : Product  Inputs=5
  p(t) : Outport
  wires:
  Clock1/1 -> Product3/5, Product1/1
  Constant3/1 -> Product1/2
  Product1/1 -> Math Function/1
  Constant4/1 -> Product3/4
  Constant1/1 -> Product3/1
  Constant2/1 -> Product3/2
  Math Function/1 -> Product3/3
  Product3/1 -> Gain/1
  Gain/1 -> p(t)/1

== system sim1S/Perturbatie p(t) new18 ==
  Clock1 : Clock
  Constant1 : Constant  Value=Dg
  Constant2 : Constant  Value=Ag
  Constant3 : Constant  Value=-1/tgM
  Constant4 : Constant  Value=1/(tgM^2)
  Gain : Gain  Gain=With_p
  Math Function : Math  SignedPower=on
  Product1 : Product
  Product3 : Product  Inputs=5
  p(t) : Outport
  wires:
  Clock1/1 -> Product3/5, Product1/1
  Constant3/1 -> Product1/2
  Product1/1 -> Math Function/1
  Constant4/1 -> Product3/4
  Constant1/1 -> Product3/1
  Constant2/1 -> Product3/2
  Math Function/1 -> Product3/3
  Product3/1 -> Gain/1
  Gain/1 -> p(t)/1

== system sim1S/Perturbatie p(t) new19 ==
  Clock1 : Clock
  Constant1 : Constant  Value=Dg
  Constant2 : Constant  Value=Ag
  Constant3 : Constant  Value=-1/tgM
  Constant4 : Constant  Value=1/(tgM^2)
  Gain : Gain  Gain=With_p
  Math Function : Math  SignedPower=on
  Product1 : Product
  Product3 : Product  Inputs=5
  p(t) : Outport
  wires:
  Clock1/1 -> Product3/5, Product1/1
  Constant3/1 -> Product1/2
  Product1/1 -> Math Function/1
  Constant4/1 -> Product3/4
  Constant1/1 -> Product3/1
  Constant2/1 -> Product3/2
  Math Function/1 -> Product3/3
  Product3/1 -> Gain/1
  Gain/1 -> p(t)/1

== system sim1S/Perturbatie p(t) new2 ==
  Clock1 : Clock
  Constant1 : Constant  Value=Dg
  Constant2 : Constant  Value=Ag
  Constant3 : Constant  Value=-1/tgM
  Constant4 : Constant  Value=1/(tgM^2)
  Gain : Gain  Gain=With_p
  Math Function : Math  SignedPower=on
  Product1 : Product
  Product3 : Product  Inputs=5
  p(t) : Outport
  wires:
  Clock1/1 -> Product3/5, Product1/1
  Constant3/1 -> Product1/2
  Product1/1 -> Math Function/1
  Constant4/1 -> Product3/4
  Constant1/1 -> Product3/1
  Constant2/1 -> Product3/2
  Math Function/1 -> Product3/3
  Product3/1 -> Gain/1
  Gain/1 -> p(t)/1

== system sim1S/Perturbatie p(t) new20 ==
  Clock1 : Clock
  Constant1 : Constant  Value=Dg
  Constant2 : Constant  Value=Ag
  Constant3 : Constant  Value=-1/tgM
  Constant4 : Constant  Value=1/(tgM^2)
  Gain : Gain  Gain=With_p
  Math Function : Math  SignedPower=on
  Product1 : Product
  Product3 : Product  Inputs=5
  p(t) : Outport
  wires:
  Clock1/1 -> Product3/5, Product1/1
  Constant3/1 -> Product1/2
  Product1/1 -> Math Function/1
  Constant4/1 -> Product3/4
  Constant1/1 -> Product3/1
  Constant2/1 -> Product3/2
  Math Function/1 -> Product3/3
  Product3/1 -> Gain/1
  Gain/1 -> p(t)/1

== system sim1S/Perturbatie p(t) new21 ==
  Clock1 : Clock
  Constant1 : Constant  Value=Dg
  Constant2 : Constant  Value=Ag
  Constant3 : Constant  Value=-1/tgM
  Constant4 : Constant  Value=1/(tgM^2)
  Gain : Gain  Gain=With_p
  Math Function : Math  SignedPower=on
  Product1 : Product
  Product3 : Product  Inputs=5
  p(t) : Outport
  wires:
  Clock1/1 -> Product3/5, Product1/1
  Constant3/1 -> Product1/2
  Product1/1 -> Math Function/1
  Constant4/1 -> Product3/4
  Constant1/1 -> Product3/1
  Constant2/1 -> Product3/2
  Math Function/1 -> Product3/3
  Product3/1 -> Gain/1
  Gain/1 -> p(t)/1

== system sim1S/Perturbatie p(t) new22 ==
  Clock1 : Clock
  Constant1 : Constant  Value=Dg
  Constant2 : Constant  Value=Ag
  Constant3 : Constant  Value=-1/tgM
  Constant4 : Constant  Value=1/(tgM^2)
  Gain : Gain  Gain=With_p
  Math Function : Math  SignedPower=on
  Product1 : Product
  Product3 : Product  Inputs=5
  p(t) : Outport
  wires:
  Clock1/1 -> Product3/5, Product1/1
  Constant3/1 -> Product1/2
  Product1/1 -> Math Function/1
  Constant4/1 -> Product3/4
  Constant1/1 -> Product3/1
  Constant2/1 -> Product3/2
  Math Function/1 -> Product3/3
  Product3/1 -> Gain/1
  Gain/1 -> p(t)/1

== system sim1S/Perturbatie p(t) new23 ==
  Clock1 : Clock
  Constant1 : Constant  Value=Dg
  Constant2 : Constant  Value=Ag
  Constant3 : Constant  Value=-1/tgM
  Constant4 : Constant  Value=1/(tgM^2)
  Gain : Gain  Gain=With_p
  Math Function : Math  SignedPower=on
  Product1 : Product
  Product3 : Product  Inputs=5
  p(t) : Outport
  wires:
  Clock1/1 -> Product3/5, Product1/1
  Constant3/1 -> Product1/2
  Product1/1 -> Math Function/1
  Constant4/1 -> Product3/4
  Constant1/1 -> Product3/1
  Constant2/1 -> Product3/2
  Math Function/1 -> Product3/3
  Product3/1 -> Gain/1
  Gain/1 -> p(t)/1
